simulink model "ModelObserver"  (R2018b)
settings: Solver=FixedStepAuto  StartTime=0.0  StopTime=200  FixedStep=0.001  RelTol=1e-3
settings Model: Creator=lexa3  LastModifiedBy=lexa3

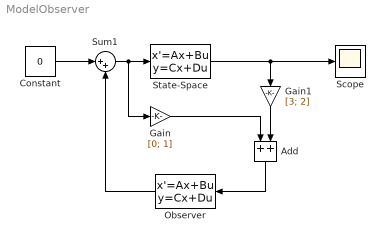
== system ModelObserver ==
  Add : Sum
  Constant : Constant  Value=0
  Gain : Gain  Gain=[0; 1]
  Gain1 : Gain  Gain=[3; 2]
  Observer : StateSpace  A=[-3 1; -2 0]  B=[1 0; 0 1]  C=[-12 -7]  D=[0 0]  InitialCondition=[0.7; 0]
  Scope : Scope
  State-Space : StateSpace  A=[0 1; 0 0]  B=[0; 1]  C=[1 0]  D=0  InitialCondition=[1; 0.001]
  Sum1 : Sum  Inputs=|++
  wires:
  Sum1/1 -> Gain/1, State-Space/1
  Constant/1 -> Sum1/1
  State-Space/1 -> Gain1/1, Scope/1
  Gain1/1 -> Add/2
  Gain/1 -> Add/1
  Add/1 -> Observer/1
  Observer/1 -> Sum1/2
